simulink model "communicatonOnly"  (R2021a)
settings: Solver=VariableStepAuto  StartTime=0.0  StopTime=10.0  RelTol=1e-3
settings Model: Creator=cyarp  LastModifiedBy=cyarp

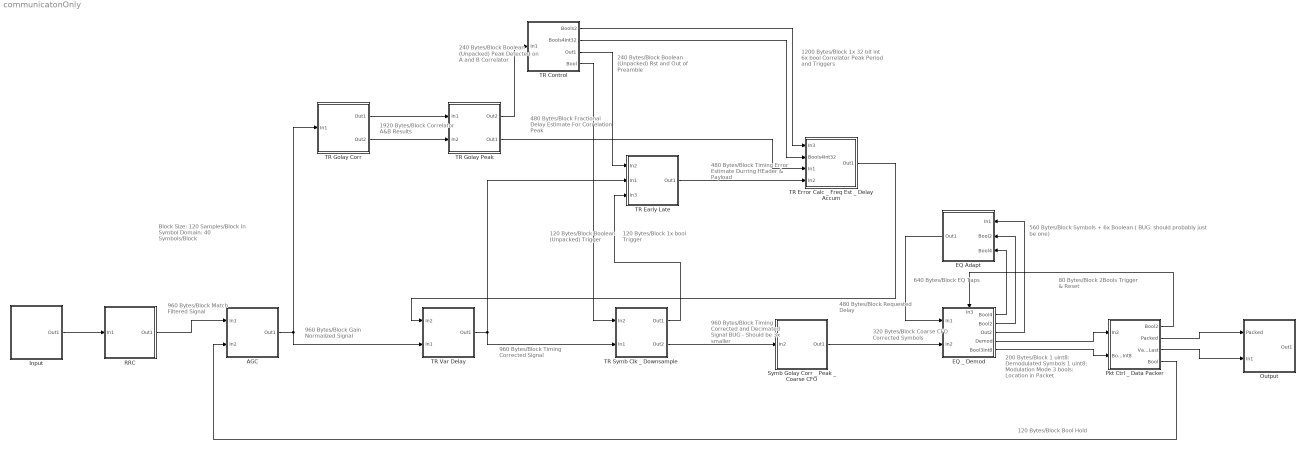
== system communicatonOnly ==
  note: 560 Bytes/Block
      | Symbols
      | + 6x Boolean ( BUG: should probably just be one)
  note: 480 Bytes/Block
      | Timing Error Estimate Durring HEader & Payload
  note: Block Size: 120 Samples/Block
      |
      | In Symbol Domain:
      | 40 Symbols/Block
  note: 960 Bytes/Block
      | Match Filtered Signal
  note: 960 Bytes/Block
      | Gain Normalized Signal
  note: 1920 Bytes/Block
      | Correlator A&B Results
  note: 480 Bytes/Block
      | Fractional Delay Estimate For Correlation Peak
  note: 480 Bytes/Block
      | Requested Delay
  note: 960 Bytes/Block
      | Timing Corrected Signal
  note: 240 Bytes/Block
      | Boolean (Unpacked)
      | Peak Detected on A and B Correlator
  note: 240 Bytes/Block
      | Boolean
      | (Unpacked)
      |
      | Rst and Out of Preamble
  note: 1200 Bytes/Block
      | 1x 32 bit int
      | 6x bool
      |
      | Correlator Peak Period and Triggers
  note: 120 Bytes/Block
      | 1x bool
      |
      | Trigger
  note: 120 Bytes/Block
      | Boolean
      | (Unpacked)
      |
      | Trigger
  note: 960 Bytes/Block
      | Timing Corrected and Decimated Signal
      |
      | BUG - Should be 3x smaller
  note: 320 Bytes/Block
      | Coarse CFO Corrected Symbols
  note: 640 Bytes/Block
      | EQ Taps
  note: 200 Bytes/Block
      | 1 uint8: Demodulated Symbols
      | 1 uint8: Modulation Mode
      | 3 bools: Location in Packet
  note: 80 Bytes/Block
      | 2Bools
      | Trigger & Reset
  note: 120 Bytes/Block
      | Bool
      | Hold
  AGC : Subsystem
  EQ Adapt : Subsystem
  EQ _ Demod : Subsystem
      settings: PortSchema="{\"entries\":[{\"content\":{\"sides\":[{\"content\":{\"connectorIds\":[\"In1\",\"In2\"]},\"type\":\"ConnectorPlacement.EquallySpacedRectSide\",\"uuid\":\"0a1b8b48-df57-4220-95fa-bccfad34cfdc\"},{\"content\":{\"connectorIds\":[\"Out1\",\"Out2\",\"Out3\",\"Out4\",\"Out5\"],\"side\":\"RIGHT\"},\"type\":\"ConnectorPlacement.EquallySpacedRectSide\",\"uuid\":\"f13a3678-3c23-4885-a146-d6be8ed5d5cd\"},{\"content\":{\"connectorIds\":[\"In3\"],\"side\":\"TOP\"},\"type\":\"ConnectorPlacement.EquallySpacedRectSide\",\"uuid\":\"f40a929f-d174-416e-9fb4-a5308a6cc714\"}]},\"type\":\"ConnectorPlacement.EquallySpacedConnector\",\"uuid\":\"75998ae4-006d-43a6-ba52-fd07b3da03f5\"}],\"packageUris\":[\"http://schema.mathworks.com/mf0/Connector/R2020b\"],\"version\":\"1.0\"}"
  Input : Subsystem
  Output : Subsystem
  Pkt Ctrl _ Data Packer : Subsystem
  RRC : Subsystem
  Symb Golay Corr _ Peak _ Coarse CFO : Subsystem
  TR Control : Subsystem
  TR Early Late : Subsystem
  TR Error Calc _ Freq Est _ Delay Accum : Subsystem
  TR Golay Corr : Subsystem
  TR Golay Peak : Subsystem
  TR Symb Clk _ Downsample : Subsystem
  TR Var Delay : Subsystem
  wires:
  RRC/1(Out1) -> AGC/1(In1)
  AGC/1(Out1) -> TR Var Delay/2(In1), TR Golay Corr/1(In1)
  TR Golay Corr/1(Out1) -> TR Golay Peak/1(In1)
  TR Golay Corr/2(Out2) -> TR Golay Peak/2(In2)
  TR Golay Peak/2(Out1) -> TR Error Calc _ Freq Est _ Delay Accum/3(In1)
  TR Error Calc _ Freq Est _ Delay Accum/1(Out1) -> TR Var Delay/1(In2)
  TR Var Delay/1(Out1) -> TR Early Late/2(In1), TR Symb Clk _ Downsample/2(In1)
  TR Early Late/1(Out1) -> TR Error Calc _ Freq Est _ Delay Accum/4(In2)
  TR Golay Peak/1(Out2) -> TR Control/1(In1)
  TR Control/3(Out1) -> TR Early Late/1(In2)
  TR Control/1(Bools2) -> TR Error Calc _ Freq Est _ Delay Accum/1(In3)
  TR Control/2(Bools4Int32) -> TR Error Calc _ Freq Est _ Delay Accum/2(Bools4Int32)
  TR Control/4(Bool) -> TR Symb Clk _ Downsample/1(In2)
  TR Symb Clk _ Downsample/1(Out1) -> TR Early Late/3(In3)
  TR Symb Clk _ Downsample/2(Out2) -> Symb Golay Corr _ Peak _ Coarse CFO/1(In2)
  Symb Golay Corr _ Peak _ Coarse CFO/1(Out1) -> EQ _ Demod/2(In2)
  EQ _ Demod/3(Out2) -> EQ Adapt/1(In1)
  EQ Adapt/1(Out1) -> EQ _ Demod/1(In1)
  EQ _ Demod/2(Bool2) -> EQ Adapt/2(Bool2)
  EQ _ Demod/1(Bool4) -> EQ Adapt/3(Bool4)
  EQ _ Demod/4(Demod) -> Pkt Ctrl _ Data Packer/1(In2)
  EQ _ Demod/5(Bool3Int8) -> Pkt Ctrl _ Data Packer/2(Bool3Int8)
  Pkt Ctrl _ Data Packer/1(Bool2) -> EQ _ Demod/3(In3)
  Pkt Ctrl _ Data Packer/3(ValidLast) -> Output/2(In1)
  Pkt Ctrl _ Data Packer/2(Packed) -> Output/1(Packed)
  Pkt Ctrl _ Data Packer/4(Bool) -> AGC/2(In2)
  Input/1(Out1) -> RRC/1(In1)

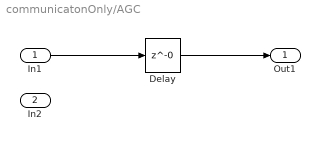
== system communicatonOnly/AGC ==
  In1 : Inport
  In2 : Inport  Port=2
  Delay : Delay  DelayLength=0
  Out1 : Outport
  wires:
  In1/1 -> Delay/1
  Delay/1 -> Out1/1

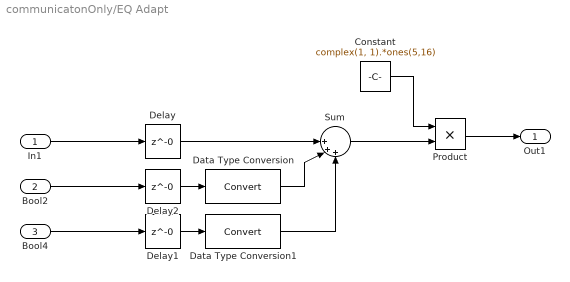
== system communicatonOnly/EQ Adapt ==
  In1 : Inport
  Bool2 : Inport  Port=2
  Bool4 : Inport  Port=3
  Constant : Constant  Value=complex(1, 1).*ones(5,16)  OutDataTypeStr=single
  Data Type Conversion : DataTypeConversion
  Data Type Conversion1 : DataTypeConversion
  Delay : Delay  DelayLength=0
  Delay1 : Delay  DelayLength=0
  Delay2 : Delay  DelayLength=0
  Product : Product  OutDataTypeStr=Inherit: Same as first input
  Sum : Sum  Inputs=||+++
  Out1 : Outport
  wires:
  In1/1 -> Delay/1
  Bool2/1 -> Delay2/1
  Bool4/1 -> Delay1/1
  Delay2/1 -> Data Type Conversion/1
  Delay1/1 -> Data Type Conversion1/1
  Delay/1 -> Sum/1
  Data Type Conversion/1 -> Sum/2
  Data Type Conversion1/1 -> Sum/3
  Sum/1 -> Product/2
  Constant/1 -> Product/1
  Product/1 -> Out1/1

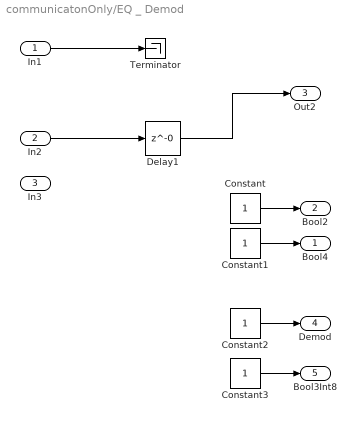
== system communicatonOnly/EQ _ Demod ==
  In1 : Inport
  In2 : Inport  Port=2
  In3 : Inport  Port=3
  Constant : Constant  OutDataTypeStr=int16
  Constant1 : Constant  OutDataTypeStr=int32
  Constant2 : Constant  OutDataTypeStr=uint8
  Constant3 : Constant  OutDataTypeStr=int32
  Delay1 : Delay  DelayLength=0
  Terminator : Terminator
  Bool4 : Outport
  Bool2 : Outport  Port=2
  Out2 : Outport  Port=3
  Demod : Outport  Port=4
  Bool3Int8 : Outport  Port=5
  wires:
  Delay1/1 -> Out2/1
  In2/1 -> Delay1/1
  Constant/1 -> Bool2/1
  Constant1/1 -> Bool4/1
  In1/1 -> Terminator/1
  Constant2/1 -> Demod/1
  Constant3/1 -> Bool3Int8/1

== system communicatonOnly/Input ==
  Constant : Constant  Value=complex(1,1)  OutDataTypeStr=single
  Out1 : Outport
  wires:
  Constant/1 -> Out1/1

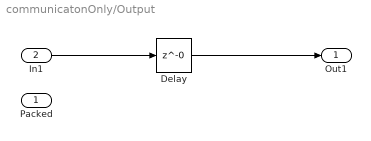
== system communicatonOnly/Output ==
  Packed : Inport
  In1 : Inport  Port=2
  Delay : Delay  DelayLength=0
  Out1 : Outport
  wires:
  In1/1 -> Delay/1
  Delay/1 -> Out1/1

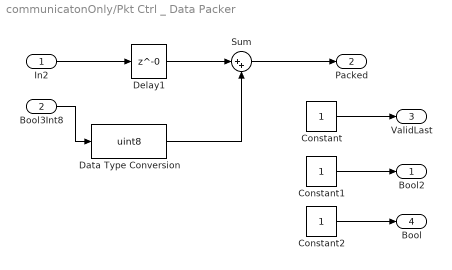
== system communicatonOnly/Pkt Ctrl _ Data Packer ==
  In2 : Inport
  Bool3Int8 : Inport  Port=2
  Constant : Constant  OutDataTypeStr=int16
  Constant1 : Constant  OutDataTypeStr=int16
  Constant2 : Constant  OutDataTypeStr=boolean
  Data Type Conversion : DataTypeConversion  OutDataTypeStr=uint8
  Delay1 : Delay  DelayLength=0
  Sum : Sum  Inputs=|++
  Bool2 : Outport
  Packed : Outport  Port=2
  ValidLast : Outport  Port=3
  Bool : Outport  Port=4
  wires:
  In2/1 -> Delay1/1
  Constant1/1 -> Bool2/1
  Constant/1 -> ValidLast/1
  Constant2/1 -> Bool/1
  Bool3Int8/1 -> Data Type Conversion/1
  Delay1/1 -> Sum/1
  Sum/1 -> Packed/1
  Data Type Conversion/1 -> Sum/2

== system communicatonOnly/RRC ==
  In1 : Inport  OutDataTypeStr=single
      settings: SignalType=complex
  Delay : Delay  DelayLength=0
  Out1 : Outport
  wires:
  In1/1 -> Delay/1
  Delay/1 -> Out1/1

== system communicatonOnly/Symb Golay Corr _ Peak _ Coarse CFO ==
  In2 : Inport
  Delay1 : Delay  DelayLength=0
  Sum : Sum  Inputs=|++
  Out1 : Outport
  wires:
  Sum/1 -> Out1/1
  In2/1 -> Delay1/1
  Delay1/1 -> Sum/1

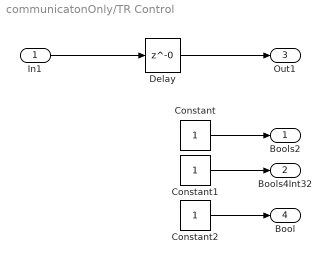
== system communicatonOnly/TR Control ==
  In1 : Inport
  Constant : Constant  OutDataTypeStr=int16
  Constant1 : Constant  OutDataTypeStr=int64
  Constant2 : Constant  OutDataTypeStr=boolean
  Delay : Delay  DelayLength=0
  Bools2 : Outport
  Bools4Int32 : Outport  Port=2
  Out1 : Outport  Port=3
  Bool : Outport  Port=4
  wires:
  In1/1 -> Delay/1
  Delay/1 -> Out1/1
  Constant/1 -> Bools2/1
  Constant1/1 -> Bools4Int32/1
  Constant2/1 -> Bool/1

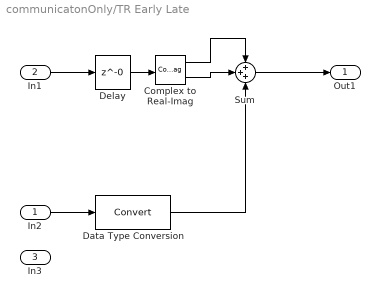
== system communicatonOnly/TR Early Late ==
  In2 : Inport
  In1 : Inport  Port=2
  In3 : Inport  Port=3
  Complex to Real-Imag : ComplexToRealImag
  Data Type Conversion : DataTypeConversion
  Delay : Delay  DelayLength=0
  Sum : Sum  Inputs=+++
  Out1 : Outport
  wires:
  In1/1 -> Delay/1
  In2/1 -> Data Type Conversion/1
  Sum/1 -> Out1/1
  Delay/1 -> Complex to Real-Imag/1
  Data Type Conversion/1 -> Sum/3
  Complex to Real-Imag/2 -> Sum/2
  Complex to Real-Imag/1 -> Sum/1

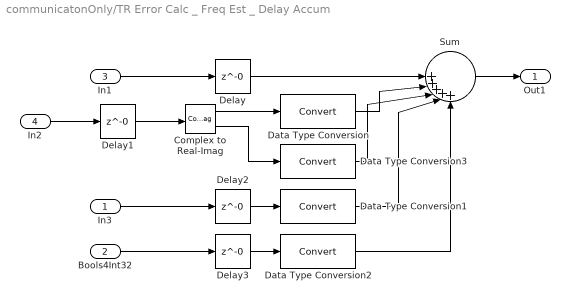
== system communicatonOnly/TR Error Calc _ Freq Est _ Delay Accum ==
  In3 : Inport
  Bools4Int32 : Inport  Port=2
  In1 : Inport  Port=3
  In2 : Inport  Port=4
  Complex to Real-Imag : ComplexToRealImag
  Data Type Conversion{,1..3} (4 alike) : DataTypeConversion
  Delay{,1..3} (4 alike) : Delay  DelayLength=0
  Sum : Sum  Inputs=||||+++++
  Out1 : Outport
  wires:
  In1/1 -> Delay/1
  In2/1 -> Delay1/1
  In3/1 -> Delay2/1
  Bools4Int32/1 -> Delay3/1
  Delay1/1 -> Complex to Real-Imag/1
  Delay2/1 -> Data Type Conversion1/1
  Delay3/1 -> Data Type Conversion2/1
  Delay/1 -> Sum/1
  Data Type Conversion/1 -> Sum/2
  Data Type Conversion1/1 -> Sum/4
  Data Type Conversion2/1 -> Sum/5
  Sum/1 -> Out1/1
  Complex to Real-Imag/1 -> Data Type Conversion/1
  Complex to Real-Imag/2 -> Data Type Conversion3/1
  Data Type Conversion3/1 -> Sum/3

== system communicatonOnly/TR Golay Corr ==
  In1 : Inport
  Delay : Delay  DelayLength=0
  Out1 : Outport
  Out2 : Outport  Port=2
  wires:
  In1/1 -> Delay/1
  Delay/1 -> Out2/1, Out1/1

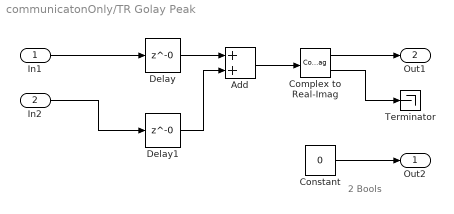
== system communicatonOnly/TR Golay Peak ==
  note: 2 Bools
  In1 : Inport
  In2 : Inport  Port=2
  Add : Sum
  Complex to Real-Imag : ComplexToRealImag
  Constant : Constant  Value=0  OutDataTypeStr=int16
  Delay : Delay  DelayLength=0
  Delay1 : Delay  DelayLength=0
  Terminator : Terminator
  Out2 : Outport
  Out1 : Outport  Port=2
  wires:
  In1/1 -> Delay/1
  In2/1 -> Delay1/1
  Delay/1 -> Add/1
  Delay1/1 -> Add/2
  Add/1 -> Complex to Real-Imag/1
  Complex to Real-Imag/1 -> Out1/1
  Complex to Real-Imag/2 -> Terminator/1
  Constant/1 -> Out2/1

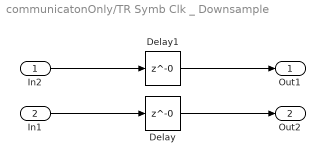
== system communicatonOnly/TR Symb Clk _ Downsample ==
  In2 : Inport
  In1 : Inport  Port=2
  Delay : Delay  DelayLength=0
  Delay1 : Delay  DelayLength=0
  Out1 : Outport
  Out2 : Outport  Port=2
  wires:
  In1/1 -> Delay/1
  In2/1 -> Delay1/1
  Delay/1 -> Out2/1
  Delay1/1 -> Out1/1

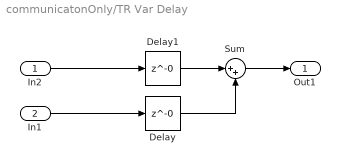
== system communicatonOnly/TR Var Delay ==
  In2 : Inport
  In1 : Inport  Port=2
  Delay : Delay  DelayLength=0
  Delay1 : Delay  DelayLength=0
  Sum : Sum  Inputs=|++
  Out1 : Outport
  wires:
  In1/1 -> Delay/1
  Sum/1 -> Out1/1
  Delay/1 -> Sum/2
  In2/1 -> Delay1/1
  Delay1/1 -> Sum/1
